simulink model "myLogPlayerProva"  (R2018a)
settings: Solver=FixedStepDiscrete  StartTime=0.0  StopTime=50000  RelTol=1e-3  EnableMultiTasking=on
undefined symbols (not defined in the file or in its folder): canChannel
libraries: canmsglib x15, canlib x3
settings Model: FPTRunName=Active  Creator=The MathWorks, Inc.  LastModifiedBy=Giovanni
settings DataIOCC: LimitDataPoints=on  SaveFormat=Array
settings OptimizationCC: BlockReduction=off  ExpressionDepthLimit=2147483647  LifeSpan=inf
settings DebuggingCC: UnderspecifiedInitializationDetection=Classic  MergeDetectMultiDrivingBlocksExec=none  SolverPrmCheckMsg=warning  FcnCallInpInsideContextMsg=warning  StateNameClashWarn=warning  SFUnexpectedBacktrackingDiag=warning  SFNoUnconditionalDefaultTransitionDiag=warning  SFExecutionAtInitializationDiag=none
settings HardwareCC: ProdBitPerPointer=32  ProdBitPerSizeT=32  ProdBitPerPtrDiffT=32  ProdLargestAtomicFloat=None  ProdIntDivRoundTo=Undefined  ProdEndianess=Unspecified  ProdWordSize=32  ProdHWDeviceType=32-bit Generic
settings ModelReferenceCC: PropagateSignalLabelsOutOfModel=off
settings RTWCC: PostCodeGenCommand=packNGo(buildInfo)  Description=Generic Real-Time Target  RetainRTWFile=on  TLCDebug=on
settings CodeAppCC: StateflowObjectComments=on
settings GRTTargetCC: TargetLangStandard=C89/C90 (ANSI)  GeneratePreprocessorConditionals=Disable all  CombineOutputUpdateFcns=off  MatFileLogging=off  GRTInterface=on
settings ConfigComp: CovMetricSettings=dw  CovHtmlReporting=on  CovSaveCumulativeToWorkspaceVar=on  CovSaveSingleToWorkspaceVar=on  CovExternalEMLEnable=off

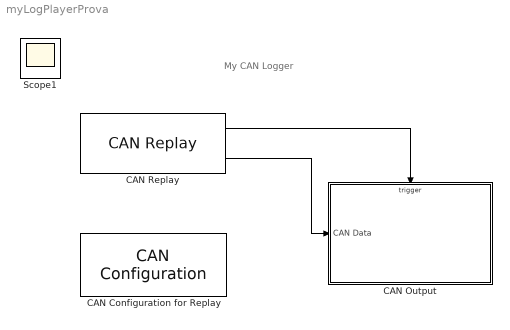
== system myLogPlayerProva ==
  note: My CAN Logger
  CAN Configuration for Replay : canlib/CAN Configuration  BlockHandle=5.0002  DeviceMenu=MathWorks Virtual 1 (Channel 1)  Device=MathWorks Virtual 1 (Channel 1)  ObjConstructor=canChannel('MathWorks', 'Virtual 1', 1)  BusSpeed=500000  EnableBitParameters=off  SJW=0  TSEG1=0  TSEG2=0  NSamples=0  AckMode=Normal
      settings: SourceProductName=Vehicle Network Toolbox  SourceProductBaseCode=VN
  CAN Output : Subsystem  TreatAsAtomicUnit=on
      settings: RTWSystemCode=Nonreusable function
  CAN Replay : canlib/CAN Replay  BlockHandle=121.0005  FullPathFileName=C:\Users\Giovanni\Documents\MATLAB\Maserati\replay.mat  FileName=replay.mat  VariableName=canMsgs  NoTimesReplay=Inf  ReplayTo=Output port  DeviceMenu=Select a device  Device=Select a device  ObjConstructor=canChannel('MathWorks','Virtual 1',1)  SampleTime=0.01  BusOutput=off
      settings: SourceProductName=Vehicle Network Toolbox  SourceProductBaseCode=VN
  Scope1 : Scope
  wires:
  CAN Replay/2 -> CAN Output/1(CAN Data)
  CAN Replay/1 -> CAN Output/Trigger

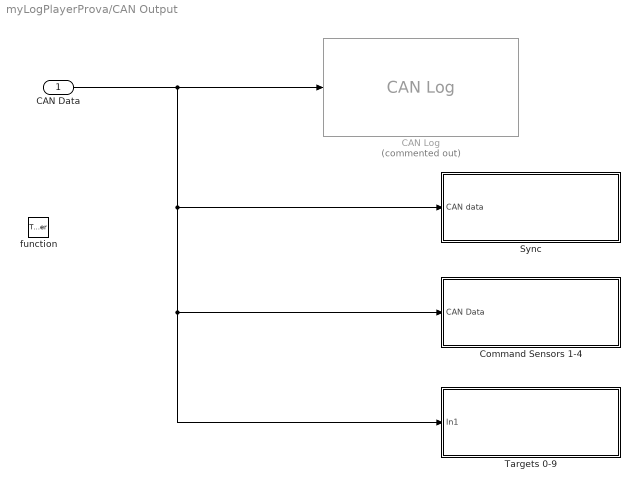
== system myLogPlayerProva/CAN Output ==
  CAN Data : Inport
  function : TriggerPort  TriggerType=function-call  VariantControl=Variant
  CAN Log : canlib/CAN Log  Commented=on  BlockHandle=12.0001  FullPathFileName=outputLog.mat  FileName=outputLog.mat  VariableName=outMsgs  MaxNumMessages=100000  LogFrom=Input port  DeviceMenu=Select a device  Device=Select a device  ObjConstructor=Select a constructor  SampleTime=0.01
      settings: SourceProductName=Vehicle Network Toolbox  SourceProductBaseCode=VN
  Command Sensors 1-4 : Subsystem  VariantControl=Variant1
  Sync : Subsystem
  Targets 0-9 : Subsystem
  wires:
  CAN Data/1 -> CAN Log/1, Sync/1(CAN data), Targets 0-9/1(In1), Command Sensors 1-4/1(CAN Data)

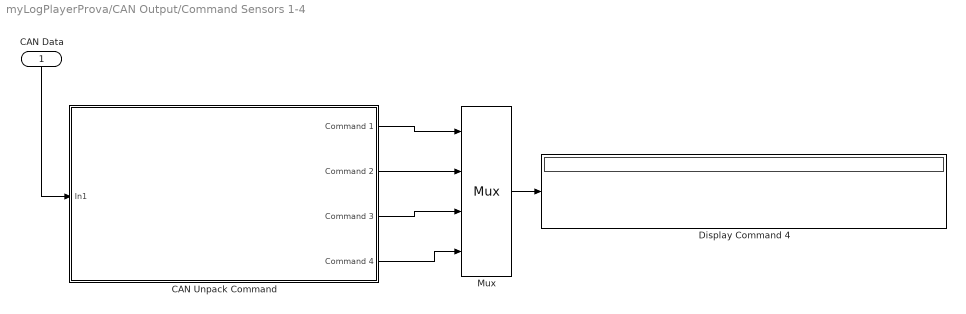
== system myLogPlayerProva/CAN Output/Command Sensors 1-4 ==
  CAN Data : Inport
  CAN Unpack Command : Subsystem
  Display Command 4 : Display
      settings: Format=hex (Stored Integer)
  Mux : Mux
  wires:
  CAN Data/1 -> CAN Unpack Command/1(In1)
  CAN Unpack Command/1(Command 1) -> Mux/1
  CAN Unpack Command/2(Command 2) -> Mux/2
  CAN Unpack Command/3(Command 3) -> Mux/3
  CAN Unpack Command/4(Command 4) -> Mux/4
  Mux/1 -> Display Command 4/1

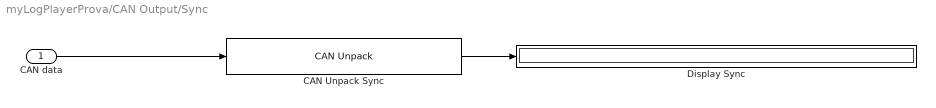
== system myLogPlayerProva/CAN Output/Sync ==
  CAN data : Inport
  CAN Unpack Sync : canmsglib/CAN Unpack  CANdbFile=VehicleInfo.dbc  MsgList=WheelSpeeds  MsgName=Sync  MsgIDType=Standard (11-bit identifier)  MsgIdentifier=hex2dec('100')  MsgLength=8  SignalInfo=LF_WSpeed$8$16$2$2$1$0$1.000000e-02$-100$0$2000$#LR_WSpeed$40$16$2$2$1$0$1.000000e-02$-100$0$2000$#RF_WSpeed$24$16$2$2$1$0$1.000000e-02$-100$0$2000$#RR_WSpeed$56$16$2$2$1$0$1.000000e-02$-100$0$2000$#  NSignals=4  IDPort=off  TimestampPort=off  ErrorPort=off  RemotePort=off  LengthPort=off  StatusPort=off  StartBits=str2num('[int32(8);int32(40);int32(24);int32(56)]')  SignalSizes=str2num('[int32(16);int32(16);int32(16);int32(16)]')  ByteOrders=str2num('[int32(2);int32(2);int32(2);int32(2)]')  DataTypes=str2num('[int32(2);int32(2);int32(2);int32(2)]')  MultiplexTypes=str2num('[int32(1);int32(1);int32(1);int32(1)]')  MultiplexValues=str2num('[double(0);double(0);double(0);double(0)]')  Factors=str2num('[double(1.000000e-02);double(1.000000e-02);double(1.000000e-02);double(1.000000e-02)]')  Offsets=str2num('[double(-100);double(-100);double(-100);double(-100)]')  Minimums=str2num('[double(0);double(0);double(0);double(0)]')  Maximums=str2num('[double(2000);double(2000);double(2000);double(2000)]')  ApplyMinMax=off
      settings: SourceProductName=Simulink Real-Time  SourceProductBaseCode=XP  DataFormat=raw data
  Display Sync : Display
      settings: Format=hex (Stored Integer)
  wires:
  CAN Unpack Sync/1 -> Display Sync/1
  CAN data/1 -> CAN Unpack Sync/1

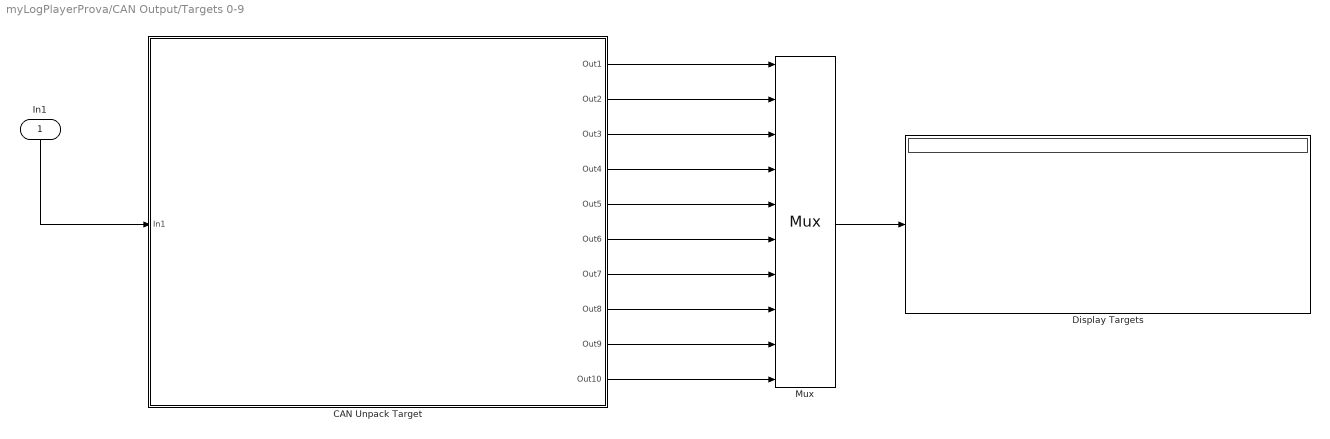
== system myLogPlayerProva/CAN Output/Targets 0-9 ==
  In1 : Inport
  CAN Unpack Target : Subsystem
  Display Targets : Display
      settings: Format=hex (Stored Integer)
  Mux : Mux  Inputs=10
  wires:
  In1/1 -> CAN Unpack Target/1(In1)
  Mux/1 -> Display Targets/1
  CAN Unpack Target/1(Out1) -> Mux/1
  CAN Unpack Target/2(Out2) -> Mux/2
  CAN Unpack Target/3(Out3) -> Mux/3
  CAN Unpack Target/4(Out4) -> Mux/4
  CAN Unpack Target/5(Out5) -> Mux/5
  CAN Unpack Target/6(Out6) -> Mux/6
  CAN Unpack Target/7(Out7) -> Mux/7
  CAN Unpack Target/8(Out8) -> Mux/8
  CAN Unpack Target/9(Out9) -> Mux/9
  CAN Unpack Target/10(Out10) -> Mux/10

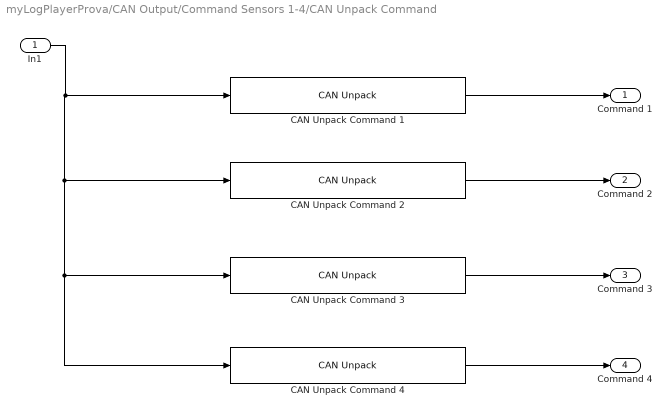
== system myLogPlayerProva/CAN Output/Command Sensors 1-4/CAN Unpack Command ==
  In1 : Inport
  CAN Unpack Command 1 : canmsglib/CAN Unpack  CANdbFile=VehicleInfo.dbc  MsgList=WheelSpeeds  MsgName=Command 1  MsgIDType=Standard (11-bit identifier)  MsgIdentifier=hex2dec('201')  MsgLength=8  SignalInfo=LF_WSpeed$8$16$2$2$1$0$1.000000e-02$-100$0$2000$#LR_WSpeed$40$16$2$2$1$0$1.000000e-02$-100$0$2000$#RF_WSpeed$24$16$2$2$1$0$1.000000e-02$-100$0$2000$#RR_WSpeed$56$16$2$2$1$0$1.000000e-02$-100$0$2000$#  NSignals=4  IDPort=off  TimestampPort=off  ErrorPort=off  RemotePort=off  LengthPort=off  StatusPort=off  StartBits=str2num('[int32(8);int32(40);int32(24);int32(56)]')  SignalSizes=str2num('[int32(16);int32(16);int32(16);int32(16)]')  ByteOrders=str2num('[int32(2);int32(2);int32(2);int32(2)]')  DataTypes=str2num('[int32(2);int32(2);int32(2);int32(2)]')  MultiplexTypes=str2num('[int32(1);int32(1);int32(1);int32(1)]')  MultiplexValues=str2num('[double(0);double(0);double(0);double(0)]')  Factors=str2num('[double(1.000000e-02);double(1.000000e-02);double(1.000000e-02);double(1.000000e-02)]')  Offsets=str2num('[double(-100);double(-100);double(-100);double(-100)]')  Minimums=str2num('[double(0);double(0);double(0);double(0)]')  Maximums=str2num('[double(2000);double(2000);double(2000);double(2000)]')  ApplyMinMax=off
      settings: SourceProductName=Simulink Real-Time  SourceProductBaseCode=XP  DataFormat=raw data
  CAN Unpack Command 2 : canmsglib/CAN Unpack  CANdbFile=VehicleInfo.dbc  MsgList=WheelSpeeds  MsgName=Command 2  MsgIDType=Standard (11-bit identifier)  MsgIdentifier=hex2dec('202')  MsgLength=8  SignalInfo=LF_WSpeed$8$16$2$2$1$0$1.000000e-02$-100$0$2000$#LR_WSpeed$40$16$2$2$1$0$1.000000e-02$-100$0$2000$#RF_WSpeed$24$16$2$2$1$0$1.000000e-02$-100$0$2000$#RR_WSpeed$56$16$2$2$1$0$1.000000e-02$-100$0$2000$#  NSignals=4  IDPort=off  TimestampPort=off  ErrorPort=off  RemotePort=off  LengthPort=off  StatusPort=off  StartBits=str2num('[int32(8);int32(40);int32(24);int32(56)]')  SignalSizes=str2num('[int32(16);int32(16);int32(16);int32(16)]')  ByteOrders=str2num('[int32(2);int32(2);int32(2);int32(2)]')  DataTypes=str2num('[int32(2);int32(2);int32(2);int32(2)]')  MultiplexTypes=str2num('[int32(1);int32(1);int32(1);int32(1)]')  MultiplexValues=str2num('[double(0);double(0);double(0);double(0)]')  Factors=str2num('[double(1.000000e-02);double(1.000000e-02);double(1.000000e-02);double(1.000000e-02)]')  Offsets=str2num('[double(-100);double(-100);double(-100);double(-100)]')  Minimums=str2num('[double(0);double(0);double(0);double(0)]')  Maximums=str2num('[double(2000);double(2000);double(2000);double(2000)]')  ApplyMinMax=off
      settings: SourceProductName=Simulink Real-Time  SourceProductBaseCode=XP  DataFormat=raw data
  CAN Unpack Command 3 : canmsglib/CAN Unpack  CANdbFile=VehicleInfo.dbc  MsgList=WheelSpeeds  MsgName=Command 3  MsgIDType=Standard (11-bit identifier)  MsgIdentifier=hex2dec('203')  MsgLength=8  SignalInfo=LF_WSpeed$8$16$2$2$1$0$1.000000e-02$-100$0$2000$#LR_WSpeed$40$16$2$2$1$0$1.000000e-02$-100$0$2000$#RF_WSpeed$24$16$2$2$1$0$1.000000e-02$-100$0$2000$#RR_WSpeed$56$16$2$2$1$0$1.000000e-02$-100$0$2000$#  NSignals=4  IDPort=off  TimestampPort=off  ErrorPort=off  RemotePort=off  LengthPort=off  StatusPort=off  StartBits=str2num('[int32(8);int32(40);int32(24);int32(56)]')  SignalSizes=str2num('[int32(16);int32(16);int32(16);int32(16)]')  ByteOrders=str2num('[int32(2);int32(2);int32(2);int32(2)]')  DataTypes=str2num('[int32(2);int32(2);int32(2);int32(2)]')  MultiplexTypes=str2num('[int32(1);int32(1);int32(1);int32(1)]')  MultiplexValues=str2num('[double(0);double(0);double(0);double(0)]')  Factors=str2num('[double(1.000000e-02);double(1.000000e-02);double(1.000000e-02);double(1.000000e-02)]')  Offsets=str2num('[double(-100);double(-100);double(-100);double(-100)]')  Minimums=str2num('[double(0);double(0);double(0);double(0)]')  Maximums=str2num('[double(2000);double(2000);double(2000);double(2000)]')  ApplyMinMax=off
      settings: SourceProductName=Simulink Real-Time  SourceProductBaseCode=XP  DataFormat=raw data
  CAN Unpack Command 4 : canmsglib/CAN Unpack  CANdbFile=VehicleInfo.dbc  MsgList=WheelSpeeds  MsgName=Command 4  MsgIDType=Standard (11-bit identifier)  MsgIdentifier=hex2dec('204')  MsgLength=8  SignalInfo=LF_WSpeed$8$16$2$2$1$0$1.000000e-02$-100$0$2000$#LR_WSpeed$40$16$2$2$1$0$1.000000e-02$-100$0$2000$#RF_WSpeed$24$16$2$2$1$0$1.000000e-02$-100$0$2000$#RR_WSpeed$56$16$2$2$1$0$1.000000e-02$-100$0$2000$#  NSignals=4  IDPort=off  TimestampPort=off  ErrorPort=off  RemotePort=off  LengthPort=off  StatusPort=off  StartBits=str2num('[int32(8);int32(40);int32(24);int32(56)]')  SignalSizes=str2num('[int32(16);int32(16);int32(16);int32(16)]')  ByteOrders=str2num('[int32(2);int32(2);int32(2);int32(2)]')  DataTypes=str2num('[int32(2);int32(2);int32(2);int32(2)]')  MultiplexTypes=str2num('[int32(1);int32(1);int32(1);int32(1)]')  MultiplexValues=str2num('[double(0);double(0);double(0);double(0)]')  Factors=str2num('[double(1.000000e-02);double(1.000000e-02);double(1.000000e-02);double(1.000000e-02)]')  Offsets=str2num('[double(-100);double(-100);double(-100);double(-100)]')  Minimums=str2num('[double(0);double(0);double(0);double(0)]')  Maximums=str2num('[double(2000);double(2000);double(2000);double(2000)]')  ApplyMinMax=off
      settings: SourceProductName=Simulink Real-Time  SourceProductBaseCode=XP  DataFormat=raw data
  Command 1 : Outport
  Command 2 : Outport  Port=2
  Command 3 : Outport  Port=3
  Command 4 : Outport  Port=4
  wires:
  In1/1 -> CAN Unpack Command 1/1, CAN Unpack Command 4/1, CAN Unpack Command 3/1, CAN Unpack Command 2/1
  CAN Unpack Command 4/1 -> Command 4/1
  CAN Unpack Command 2/1 -> Command 2/1
  CAN Unpack Command 3/1 -> Command 3/1
  CAN Unpack Command 1/1 -> Command 1/1

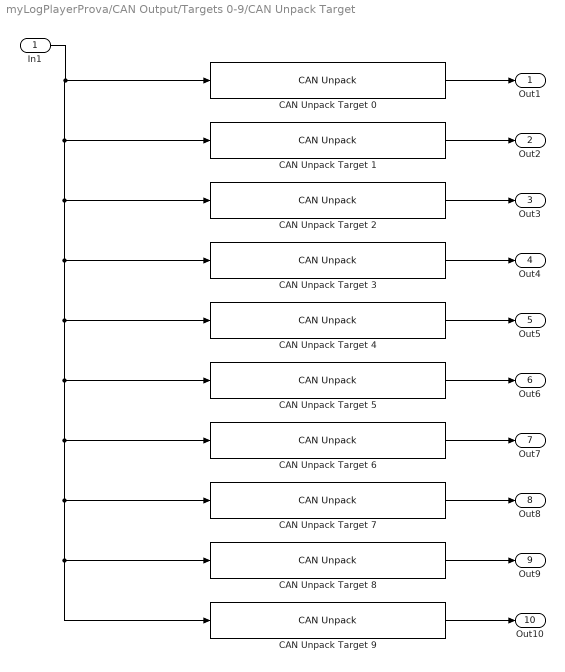
== system myLogPlayerProva/CAN Output/Targets 0-9/CAN Unpack Target ==
  In1 : Inport
  CAN Unpack Target 0 : canmsglib/CAN Unpack  CANdbFile=VehicleInfo.dbc  MsgList=WheelSpeeds  MsgName=Target 0  MsgIDType=Standard (11-bit identifier)  MsgIdentifier=hex2dec('300')  MsgLength=8  SignalInfo=LF_WSpeed$8$16$2$2$1$0$1.000000e-02$-100$0$2000$#LR_WSpeed$40$16$2$2$1$0$1.000000e-02$-100$0$2000$#RF_WSpeed$24$16$2$2$1$0$1.000000e-02$-100$0$2000$#RR_WSpeed$56$16$2$2$1$0$1.000000e-02$-100$0$2000$#  NSignals=4  IDPort=off  TimestampPort=off  ErrorPort=off  RemotePort=off  LengthPort=off  StatusPort=off  StartBits=str2num('[int32(8);int32(40);int32(24);int32(56)]')  SignalSizes=str2num('[int32(16);int32(16);int32(16);int32(16)]')  ByteOrders=str2num('[int32(2);int32(2);int32(2);int32(2)]')  DataTypes=str2num('[int32(2);int32(2);int32(2);int32(2)]')  MultiplexTypes=str2num('[int32(1);int32(1);int32(1);int32(1)]')  MultiplexValues=str2num('[double(0);double(0);double(0);double(0)]')  Factors=str2num('[double(1.000000e-02);double(1.000000e-02);double(1.000000e-02);double(1.000000e-02)]')  Offsets=str2num('[double(-100);double(-100);double(-100);double(-100)]')  Minimums=str2num('[double(0);double(0);double(0);double(0)]')  Maximums=str2num('[double(2000);double(2000);double(2000);double(2000)]')  ApplyMinMax=off
      settings: SourceProductName=Simulink Real-Time  SourceProductBaseCode=XP  DataFormat=raw data
  CAN Unpack Target 1 : canmsglib/CAN Unpack  CANdbFile=VehicleInfo.dbc  MsgList=WheelSpeeds  MsgName=Target 1  MsgIDType=Standard (11-bit identifier)  MsgIdentifier=hex2dec('301')  MsgLength=8  SignalInfo=LF_WSpeed$8$16$2$2$1$0$1.000000e-02$-100$0$2000$#LR_WSpeed$40$16$2$2$1$0$1.000000e-02$-100$0$2000$#RF_WSpeed$24$16$2$2$1$0$1.000000e-02$-100$0$2000$#RR_WSpeed$56$16$2$2$1$0$1.000000e-02$-100$0$2000$#  NSignals=4  IDPort=off  TimestampPort=off  ErrorPort=off  RemotePort=off  LengthPort=off  StatusPort=off  StartBits=str2num('[int32(8);int32(40);int32(24);int32(56)]')  SignalSizes=str2num('[int32(16);int32(16);int32(16);int32(16)]')  ByteOrders=str2num('[int32(2);int32(2);int32(2);int32(2)]')  DataTypes=str2num('[int32(2);int32(2);int32(2);int32(2)]')  MultiplexTypes=str2num('[int32(1);int32(1);int32(1);int32(1)]')  MultiplexValues=str2num('[double(0);double(0);double(0);double(0)]')  Factors=str2num('[double(1.000000e-02);double(1.000000e-02);double(1.000000e-02);double(1.000000e-02)]')  Offsets=str2num('[double(-100);double(-100);double(-100);double(-100)]')  Minimums=str2num('[double(0);double(0);double(0);double(0)]')  Maximums=str2num('[double(2000);double(2000);double(2000);double(2000)]')  ApplyMinMax=off
      settings: SourceProductName=Simulink Real-Time  SourceProductBaseCode=XP  DataFormat=raw data
  CAN Unpack Target 2 : canmsglib/CAN Unpack  CANdbFile=VehicleInfo.dbc  MsgList=WheelSpeeds  MsgName=Target 2  MsgIDType=Standard (11-bit identifier)  MsgIdentifier=hex2dec('302')  MsgLength=8  SignalInfo=LF_WSpeed$8$16$2$2$1$0$1.000000e-02$-100$0$2000$#LR_WSpeed$40$16$2$2$1$0$1.000000e-02$-100$0$2000$#RF_WSpeed$24$16$2$2$1$0$1.000000e-02$-100$0$2000$#RR_WSpeed$56$16$2$2$1$0$1.000000e-02$-100$0$2000$#  NSignals=4  IDPort=off  TimestampPort=off  ErrorPort=off  RemotePort=off  LengthPort=off  StatusPort=off  StartBits=str2num('[int32(8);int32(40);int32(24);int32(56)]')  SignalSizes=str2num('[int32(16);int32(16);int32(16);int32(16)]')  ByteOrders=str2num('[int32(2);int32(2);int32(2);int32(2)]')  DataTypes=str2num('[int32(2);int32(2);int32(2);int32(2)]')  MultiplexTypes=str2num('[int32(1);int32(1);int32(1);int32(1)]')  MultiplexValues=str2num('[double(0);double(0);double(0);double(0)]')  Factors=str2num('[double(1.000000e-02);double(1.000000e-02);double(1.000000e-02);double(1.000000e-02)]')  Offsets=str2num('[double(-100);double(-100);double(-100);double(-100)]')  Minimums=str2num('[double(0);double(0);double(0);double(0)]')  Maximums=str2num('[double(2000);double(2000);double(2000);double(2000)]')  ApplyMinMax=off
      settings: SourceProductName=Simulink Real-Time  SourceProductBaseCode=XP  DataFormat=raw data
  CAN Unpack Target 3 : canmsglib/CAN Unpack  CANdbFile=VehicleInfo.dbc  MsgList=WheelSpeeds  MsgName=Target 3  MsgIDType=Standard (11-bit identifier)  MsgIdentifier=hex2dec('303')  MsgLength=8  SignalInfo=LF_WSpeed$8$16$2$2$1$0$1.000000e-02$-100$0$2000$#LR_WSpeed$40$16$2$2$1$0$1.000000e-02$-100$0$2000$#RF_WSpeed$24$16$2$2$1$0$1.000000e-02$-100$0$2000$#RR_WSpeed$56$16$2$2$1$0$1.000000e-02$-100$0$2000$#  NSignals=4  IDPort=off  TimestampPort=off  ErrorPort=off  RemotePort=off  LengthPort=off  StatusPort=off  StartBits=str2num('[int32(8);int32(40);int32(24);int32(56)]')  SignalSizes=str2num('[int32(16);int32(16);int32(16);int32(16)]')  ByteOrders=str2num('[int32(2);int32(2);int32(2);int32(2)]')  DataTypes=str2num('[int32(2);int32(2);int32(2);int32(2)]')  MultiplexTypes=str2num('[int32(1);int32(1);int32(1);int32(1)]')  MultiplexValues=str2num('[double(0);double(0);double(0);double(0)]')  Factors=str2num('[double(1.000000e-02);double(1.000000e-02);double(1.000000e-02);double(1.000000e-02)]')  Offsets=str2num('[double(-100);double(-100);double(-100);double(-100)]')  Minimums=str2num('[double(0);double(0);double(0);double(0)]')  Maximums=str2num('[double(2000);double(2000);double(2000);double(2000)]')  ApplyMinMax=off
      settings: SourceProductName=Simulink Real-Time  SourceProductBaseCode=XP  DataFormat=raw data
  CAN Unpack Target 4 : canmsglib/CAN Unpack  CANdbFile=VehicleInfo.dbc  MsgList=WheelSpeeds  MsgName=Target 4  MsgIDType=Standard (11-bit identifier)  MsgIdentifier=hex2dec('304')  MsgLength=8  SignalInfo=LF_WSpeed$8$16$2$2$1$0$1.000000e-02$-100$0$2000$#LR_WSpeed$40$16$2$2$1$0$1.000000e-02$-100$0$2000$#RF_WSpeed$24$16$2$2$1$0$1.000000e-02$-100$0$2000$#RR_WSpeed$56$16$2$2$1$0$1.000000e-02$-100$0$2000$#  NSignals=4  IDPort=off  TimestampPort=off  ErrorPort=off  RemotePort=off  LengthPort=off  StatusPort=off  StartBits=str2num('[int32(8);int32(40);int32(24);int32(56)]')  SignalSizes=str2num('[int32(16);int32(16);int32(16);int32(16)]')  ByteOrders=str2num('[int32(2);int32(2);int32(2);int32(2)]')  DataTypes=str2num('[int32(2);int32(2);int32(2);int32(2)]')  MultiplexTypes=str2num('[int32(1);int32(1);int32(1);int32(1)]')  MultiplexValues=str2num('[double(0);double(0);double(0);double(0)]')  Factors=str2num('[double(1.000000e-02);double(1.000000e-02);double(1.000000e-02);double(1.000000e-02)]')  Offsets=str2num('[double(-100);double(-100);double(-100);double(-100)]')  Minimums=str2num('[double(0);double(0);double(0);double(0)]')  Maximums=str2num('[double(2000);double(2000);double(2000);double(2000)]')  ApplyMinMax=off
      settings: SourceProductName=Simulink Real-Time  SourceProductBaseCode=XP  DataFormat=raw data
  CAN Unpack Target 5 : canmsglib/CAN Unpack  CANdbFile=VehicleInfo.dbc  MsgList=WheelSpeeds  MsgName=Target 5  MsgIDType=Standard (11-bit identifier)  MsgIdentifier=hex2dec('305')  MsgLength=8  SignalInfo=LF_WSpeed$8$16$2$2$1$0$1.000000e-02$-100$0$2000$#LR_WSpeed$40$16$2$2$1$0$1.000000e-02$-100$0$2000$#RF_WSpeed$24$16$2$2$1$0$1.000000e-02$-100$0$2000$#RR_WSpeed$56$16$2$2$1$0$1.000000e-02$-100$0$2000$#  NSignals=4  IDPort=off  TimestampPort=off  ErrorPort=off  RemotePort=off  LengthPort=off  StatusPort=off  StartBits=str2num('[int32(8);int32(40);int32(24);int32(56)]')  SignalSizes=str2num('[int32(16);int32(16);int32(16);int32(16)]')  ByteOrders=str2num('[int32(2);int32(2);int32(2);int32(2)]')  DataTypes=str2num('[int32(2);int32(2);int32(2);int32(2)]')  MultiplexTypes=str2num('[int32(1);int32(1);int32(1);int32(1)]')  MultiplexValues=str2num('[double(0);double(0);double(0);double(0)]')  Factors=str2num('[double(1.000000e-02);double(1.000000e-02);double(1.000000e-02);double(1.000000e-02)]')  Offsets=str2num('[double(-100);double(-100);double(-100);double(-100)]')  Minimums=str2num('[double(0);double(0);double(0);double(0)]')  Maximums=str2num('[double(2000);double(2000);double(2000);double(2000)]')  ApplyMinMax=off
      settings: SourceProductName=Simulink Real-Time  SourceProductBaseCode=XP  DataFormat=raw data
  CAN Unpack Target 6 : canmsglib/CAN Unpack  CANdbFile=VehicleInfo.dbc  MsgList=WheelSpeeds  MsgName=Target 6  MsgIDType=Standard (11-bit identifier)  MsgIdentifier=hex2dec('306')  MsgLength=8  SignalInfo=LF_WSpeed$8$16$2$2$1$0$1.000000e-02$-100$0$2000$#LR_WSpeed$40$16$2$2$1$0$1.000000e-02$-100$0$2000$#RF_WSpeed$24$16$2$2$1$0$1.000000e-02$-100$0$2000$#RR_WSpeed$56$16$2$2$1$0$1.000000e-02$-100$0$2000$#  NSignals=4  IDPort=off  TimestampPort=off  ErrorPort=off  RemotePort=off  LengthPort=off  StatusPort=off  StartBits=str2num('[int32(8);int32(40);int32(24);int32(56)]')  SignalSizes=str2num('[int32(16);int32(16);int32(16);int32(16)]')  ByteOrders=str2num('[int32(2);int32(2);int32(2);int32(2)]')  DataTypes=str2num('[int32(2);int32(2);int32(2);int32(2)]')  MultiplexTypes=str2num('[int32(1);int32(1);int32(1);int32(1)]')  MultiplexValues=str2num('[double(0);double(0);double(0);double(0)]')  Factors=str2num('[double(1.000000e-02);double(1.000000e-02);double(1.000000e-02);double(1.000000e-02)]')  Offsets=str2num('[double(-100);double(-100);double(-100);double(-100)]')  Minimums=str2num('[double(0);double(0);double(0);double(0)]')  Maximums=str2num('[double(2000);double(2000);double(2000);double(2000)]')  ApplyMinMax=off
      settings: SourceProductName=Simulink Real-Time  SourceProductBaseCode=XP  DataFormat=raw data
  CAN Unpack Target 7 : canmsglib/CAN Unpack  CANdbFile=VehicleInfo.dbc  MsgList=WheelSpeeds  MsgName=Target 7  MsgIDType=Standard (11-bit identifier)  MsgIdentifier=hex2dec('307')  MsgLength=8  SignalInfo=LF_WSpeed$8$16$2$2$1$0$1.000000e-02$-100$0$2000$#LR_WSpeed$40$16$2$2$1$0$1.000000e-02$-100$0$2000$#RF_WSpeed$24$16$2$2$1$0$1.000000e-02$-100$0$2000$#RR_WSpeed$56$16$2$2$1$0$1.000000e-02$-100$0$2000$#  NSignals=4  IDPort=off  TimestampPort=off  ErrorPort=off  RemotePort=off  LengthPort=off  StatusPort=off  StartBits=str2num('[int32(8);int32(40);int32(24);int32(56)]')  SignalSizes=str2num('[int32(16);int32(16);int32(16);int32(16)]')  ByteOrders=str2num('[int32(2);int32(2);int32(2);int32(2)]')  DataTypes=str2num('[int32(2);int32(2);int32(2);int32(2)]')  MultiplexTypes=str2num('[int32(1);int32(1);int32(1);int32(1)]')  MultiplexValues=str2num('[double(0);double(0);double(0);double(0)]')  Factors=str2num('[double(1.000000e-02);double(1.000000e-02);double(1.000000e-02);double(1.000000e-02)]')  Offsets=str2num('[double(-100);double(-100);double(-100);double(-100)]')  Minimums=str2num('[double(0);double(0);double(0);double(0)]')  Maximums=str2num('[double(2000);double(2000);double(2000);double(2000)]')  ApplyMinMax=off
      settings: SourceProductName=Simulink Real-Time  SourceProductBaseCode=XP  DataFormat=raw data
  CAN Unpack Target 8 : canmsglib/CAN Unpack  CANdbFile=VehicleInfo.dbc  MsgList=WheelSpeeds  MsgName=Target 8  MsgIDType=Standard (11-bit identifier)  MsgIdentifier=hex2dec('308')  MsgLength=8  SignalInfo=LF_WSpeed$8$16$2$2$1$0$1.000000e-02$-100$0$2000$#LR_WSpeed$40$16$2$2$1$0$1.000000e-02$-100$0$2000$#RF_WSpeed$24$16$2$2$1$0$1.000000e-02$-100$0$2000$#RR_WSpeed$56$16$2$2$1$0$1.000000e-02$-100$0$2000$#  NSignals=4  IDPort=off  TimestampPort=off  ErrorPort=off  RemotePort=off  LengthPort=off  StatusPort=off  StartBits=str2num('[int32(8);int32(40);int32(24);int32(56)]')  SignalSizes=str2num('[int32(16);int32(16);int32(16);int32(16)]')  ByteOrders=str2num('[int32(2);int32(2);int32(2);int32(2)]')  DataTypes=str2num('[int32(2);int32(2);int32(2);int32(2)]')  MultiplexTypes=str2num('[int32(1);int32(1);int32(1);int32(1)]')  MultiplexValues=str2num('[double(0);double(0);double(0);double(0)]')  Factors=str2num('[double(1.000000e-02);double(1.000000e-02);double(1.000000e-02);double(1.000000e-02)]')  Offsets=str2num('[double(-100);double(-100);double(-100);double(-100)]')  Minimums=str2num('[double(0);double(0);double(0);double(0)]')  Maximums=str2num('[double(2000);double(2000);double(2000);double(2000)]')  ApplyMinMax=off
      settings: SourceProductName=Simulink Real-Time  SourceProductBaseCode=XP  DataFormat=raw data
  CAN Unpack Target 9 : canmsglib/CAN Unpack  CANdbFile=VehicleInfo.dbc  MsgList=WheelSpeeds  MsgName=Target 9  MsgIDType=Standard (11-bit identifier)  MsgIdentifier=hex2dec('309')  MsgLength=8  SignalInfo=LF_WSpeed$8$16$2$2$1$0$1.000000e-02$-100$0$2000$#LR_WSpeed$40$16$2$2$1$0$1.000000e-02$-100$0$2000$#RF_WSpeed$24$16$2$2$1$0$1.000000e-02$-100$0$2000$#RR_WSpeed$56$16$2$2$1$0$1.000000e-02$-100$0$2000$#  NSignals=4  IDPort=off  TimestampPort=off  ErrorPort=off  RemotePort=off  LengthPort=off  StatusPort=off  StartBits=str2num('[int32(8);int32(40);int32(24);int32(56)]')  SignalSizes=str2num('[int32(16);int32(16);int32(16);int32(16)]')  ByteOrders=str2num('[int32(2);int32(2);int32(2);int32(2)]')  DataTypes=str2num('[int32(2);int32(2);int32(2);int32(2)]')  MultiplexTypes=str2num('[int32(1);int32(1);int32(1);int32(1)]')  MultiplexValues=str2num('[double(0);double(0);double(0);double(0)]')  Factors=str2num('[double(1.000000e-02);double(1.000000e-02);double(1.000000e-02);double(1.000000e-02)]')  Offsets=str2num('[double(-100);double(-100);double(-100);double(-100)]')  Minimums=str2num('[double(0);double(0);double(0);double(0)]')  Maximums=str2num('[double(2000);double(2000);double(2000);double(2000)]')  ApplyMinMax=off
      settings: SourceProductName=Simulink Real-Time  SourceProductBaseCode=XP  DataFormat=raw data
  Out1 : Outport
  Out2 : Outport  Port=2
  Out3 : Outport  Port=3
  Out4 : Outport  Port=4
  Out5 : Outport  Port=5
  Out6 : Outport  Port=6
  Out7 : Outport  Port=7
  Out8 : Outport  Port=8
  Out9 : Outport  Port=9
  Out10 : Outport  Port=10
  wires:
  In1/1 -> CAN Unpack Target 0/1, CAN Unpack Target 9/1, CAN Unpack Target 8/1, CAN Unpack Target 7/1, CAN Unpack Target 6/1, CAN Unpack Target 5/1, CAN Unpack Target 4/1, CAN Unpack Target 3/1, CAN Unpack Target 2/1, CAN Unpack Target 1/1
  CAN Unpack Target 3/1 -> Out4/1
  CAN Unpack Target 8/1 -> Out9/1
  CAN Unpack Target 2/1 -> Out3/1
  CAN Unpack Target 1/1 -> Out2/1
  CAN Unpack Target 4/1 -> Out5/1
  CAN Unpack Target 5/1 -> Out6/1
  CAN Unpack Target 7/1 -> Out8/1
  CAN Unpack Target 6/1 -> Out7/1
  CAN Unpack Target 0/1 -> Out1/1
  CAN Unpack Target 9/1 -> Out10/1
